simulink model "SimTest"  (R2019b)
settings: Solver=ode45  StartTime=0.0  StopTime=20  MaxStep=0.01  RelTol=1e-3  EnableMultiTasking=on
model workspace: external: MATLAB File sm_welding_robot_params.m (data not in the file)
values from neighbouring files (symbols this model uses):
  m = [6.25, 5, 1.25, 0.9817, 1.25, 0.125]    [ImprovedApproachLawSMC.m]    (also in Puma560CaneModel.m = [0, 17.4, 4.8, 0.82, 0.34, 0.09])
  N = N + m(i)*(cell2mat(W)*VT{i}'*(dVT{i}*cell2mat(WT')+VT{i}*cell2mat(dWT')))+W{i}*J{i}*dWT{i}+W{i}*WTdth{i}*J{i}*WT{i}    [ImprovedApproachLawSMC.m]    (also in Puma560CaneModel.m)
  s = c.*e + de    [ImprovedApproachLawSMC.m]
undefined symbols (not defined in the file or in its folder): color, density, path, robot, workpiece, X, Y, Z
libraries: sm_lib x63, nesl_utility x13, sm_welding_robot_lib x7
(part 1 of 2)
Description:
  | Computing Actuator Torques Using Inverse Dynamics
  | 
  | This example illustrates the use of motion actuation to determine the actuator torques needed for the robot to achieve a given welding task.
  | The system consists of a seven degree of freedom robot carrying a welding torch. The tip of the torch needs to trace the joints being welded. In
  | this example the tip of the torch is made to trace (using motion actuation) a plus sign, a circle and a star sign on the workpiece. The torch is
  | lifted off the workpiece when transitioning between the different shapes. The motion of the welding torch is specified and the actuator
  | torques required at the various joints of the robot to achieve this motion is computed.
settings Model: Creator=MathWorks  LastModifiedBy=Priscilla
settings DataIOCC: LimitDataPoints=on  SaveFormat=Array  SaveOutput=off  SaveTime=off  ReturnWorkspaceOutputs=off
settings OptimizationCC: LifeSpan=inf
settings DebuggingCC: UnderspecifiedInitializationDetection=Classic  MergeDetectMultiDrivingBlocksExec=none  SFUnexpectedBacktrackingDiag=warning  SFNoUnconditionalDefaultTransitionDiag=warning  SFExecutionAtInitializationDiag=none  ArithmeticOperatorsInVariantConditions=warning
settings HardwareCC: ProdBitPerPointer=32  ProdBitPerSizeT=32  ProdBitPerPtrDiffT=32  ProdLargestAtomicFloat=None  ProdIntDivRoundTo=Undefined  ProdEndianess=Unspecified  ProdWordSize=32  ProdHWDeviceType=32-bit Generic
settings ModelReferenceCC: PropagateSignalLabelsOutOfModel=off
settings SFSimCC: SimUseLocalCustomCode=off  CustomCodeUndefinedFunction=UseInterfaceOnly
settings RTWCC: RTWUseLocalCustomCode=off
settings CodeAppCC: StateflowObjectComments=on
settings GRTTargetCC: TargetLangStandard=C89/C90 (ANSI)  GeneratePreprocessorConditionals=Disable all
settings ConfigComp: CovMetricSettings=dw  CovHtmlReporting=on  CovSaveCumulativeToWorkspaceVar=on  CovSaveSingleToWorkspaceVar=on  CovExternalEMLEnable=off  CovSFcnEnable=off
settings SimscapeCC: SimscapeNormalizeSystem=off
settings ConfigurationSet: Description=SimMechanics 2G
settings DiagnosticsConfigSet: SimMechanicsUnconnectedFramePorts=none
settings ExplorerConfigSet: InternalSimMechanicsExplorerSettings="<ExplorerConfiguration><canonicalview>default</canonicalview><TilePanel><TileInfo><Tiles Columns=\"1\" Count=\"1\" Rows=\"1\"><Column Left=\"2\" Weight=\"1\"/><Column Left=\"702\"/><Row Top=\"2\" Weight=\"1\"/><Row Top=\"609\"/><Tile Height=\"1\" Width=\"1\" X=\"0\" Y=\"0\"/></Tiles></TileInfo><SceneInfo><SceneViewer><BGColor><R>0.60000002384185791</R><G>0.60000002384185791</G><B>0.60000002384185791</B></BGColor><Camera><Position><X>2.70313193911561722</X><Y>-2.01174652149009159</Y><Z>3.03337065647681836</Z></Position><Center><X>0.60321557915254076</X><Y>0.0881698384729807105</Y><Z>0.933454296513737347</Z></Center><Up><X>-0.408248290463863073</X><Y>0.408248290463863073</Y><Z>0.816496580927726145</Z></Up><Left>-0.59695774513732025</Left><Right>0.59695774513732025</Right><Bottom>-0.82465145012954455</Bottom><Top>0.82465145012954455</Top></Camera></SceneViewer></SceneInfo></TilePanel></ExplorerConfiguration>"

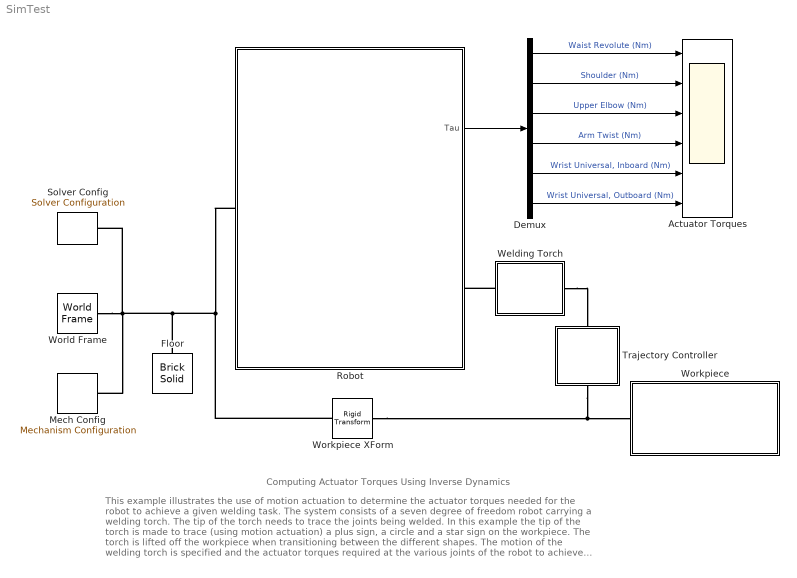
== system SimTest ==
  note: Computing Actuator Torques Using Inverse Dynamics
  note: This example illustrates the use of motion actuation to determine the actuator torques needed for the robot to achieve a given welding task.
      | The system consists of a seven degree of freedom robot carrying a welding torch. The tip of the torch needs to trace the joints being welded.
      | In this example the tip of the torch is made to trace (using motion actuation) a plus sign, a circle and a star sign on the workpiece. The torch is
      | lifted off the workpiece when transitioning between the different shapes. The motion of the welding torch is specified and the actuator torques
      | required at the various joints of the robot to achieve this motion are computed.
  Actuator Torques : Scope  NumInputPorts=6
  Demux : Demux  Outputs=6
  Floor : sm_lib/Body Elements/Brick Solid  GraphicAmbientColor=[0.15 0.15 0.15 1.0]  BasedOnType=Density  BrickDimensions=[floor.length floor.width floor.thickness]  BrickDimensionUnits=cm  CenterOfMass=[0 0 0]  CenterOfMassUnits=m  GraphicDiffuseColor=color.grey  Density=density.aluminum  DensityUnits=kg/(m^3)  DoExposeReferenceFrame=on  GraphicEmissiveColor=[0.0 0.0 0.0 1.0]  ExportEntireGeometry=off  SerializedFrames=<Frames/>  MarkerShape=Sphere  MarkerSize=10  GraphicType=FromGeometry  InertiaType=CalculateFromGeometry  Mass=1  MassUnits=kg  MomentsOfInertia=[1 1 1]  MomentsOfInertiaUnits=kg*m^2  GraphicOpacity=0.5  ProductsOfInertia=[0 0 0]  ProductsOfInertiaUnits=kg*m^2  GraphicShininess=75  GraphicSpecularColor=[0.5 0.5 0.5 1.0]  GraphicVisPropType=SimpleVisualProperties
  Mech Config : sm_lib/Utilities/Mechanism Configuration  UniformGravity=Constant  GravityVector=[0 0 -9.80665]  GravityUnits=m/s^2  LinearizationDelta=0.001
  Robot : Subsystem
      mask Display:
      | image(imread(fullfile(matlabroot,'toolbox','physmod','sm','smdemos','welding_robot','images','sm_wrobot_robot.png')));
      | port_label('RConn',1,'Tool')
      | port_label('LConn',1,'Floor')
      | port_label('output',1,'Tau')
  Solver Config : nesl_utility/Solver Configuration  PhysicalDomain=network_engine_domain  SubClassName=solver  LeftPortType=input  RightPortType=generic  Tones=[]  Harmonics=[]  SimulateNoise=off  Profile=off  UseLocalSampling=off  EnableSwitchedLinearOptims=on  FrequencyDomain=off  UseCCode=off  RelTol=0.001  AbsTol=1e-06  MinStep=1e-09  ToWorkspace=off  RevertToSquareIcSolve=off  NumHomotopyIterations=100  PhasorMode=off  PhasorModeNumHarmonics=1  DoDC=off  ResidualTolerance=1e-09  UseLocalSolver=off  LocalSolverChoice=NE_BACKWARD_EULER_ADVANCER  LocalSolverSampleTime=0.001  DoFixedCost=off  MaxNonlinIter=3  MaxModeIter=2  LinearAlgebra=Sparse  EquationFormulation=NE_TIME_EF  DelaysMemoryBudget=1024  AutomaticFiltering=on  FilteringTimeConstant=0.001  PartitionStorageMethod=AS_NEEDED  PartitionMemoryBudget=1024  PartitionMethod=FAST
  Trajectory Controller : Subsystem  mask(Trajectory Controller){tool_home=workpiece.tool.home, z_off=workpiece.tool.zoffset, glyph_sep=workpiece.glyphsep, plus_arm=workpiece.plus.armlength, circle_radius=workpiece.circle.radius, star_radius=workpiece.star.radius}
      mask prompts: tool_home "Tool Home (cm)"; z_off "Tool Off Distance (cm)"; glyph_sep "Glyph Separation (cm)"; plus_arm "Plus arm length (cm)"; circle_radius "Circle radius (cm)"; star_radius "Star circumcircle radius (cm)"
      mask help: This block controls the position and orientation of the follower frame (F) with respect to the base frame (B).
      mask init:
      | % Start tool path in home configuration
      | tool_path = [...
      |     0 tool_home'; ...
      |     1 tool_home'; ...
      |     ];
      | 
      | % Plus
      | plus = [ ...
      |     0   0 plus_arm/2 z_off; ...
      |     0.2 0 plus_arm/2 z_off; ...
      |     0.6 0 plus_arm/2 0; ...
      |     2.2 0 -plus_arm/2 0; ...
      |     2.6 -plus_arm/2 0 z_off; ...
      |     3   -plus_arm/2 0 0; ...
      |     4.6 +plus_arm/2 0 0; ...
      |     5   +plus_arm/2 0 z_off; ...
      |     ];
      | plus(:,2) = plus(:,2) - glyph_sep;
      | plus(:,1) = plus(:,1) + tool_path(end, 1) + 1;
      | tool_path = [tool_path; plus];
      | 
      | % Circle
      | dt = 3;
      | theta = (90:1:450)' * pi/180;
      | n = size(theta, 1);
      | pts = circle_radius * [cos(theta), sin(theta)];
      | circle = [ ...
      |     0 0 circle_radius z_off; ...
      |     linspace(0.4, 0.4 + dt, n)', pts, zeros(n, 1); ...
      |     (0.8 + dt) 0 circle_radius z_off; ...
      |     ];
      | circle(:,1) = circle(:,1) + tool_path(end, 1) + 1;
      | tool_path = [tool_path; circle];
      | 
      | % Star
      | dt = 3;
      | theta = (90:144:810)' * pi/180;
      | pts = star_radius * [cos(theta), sin(theta)];
      | star = [ ...
      |     0 0 star_radius z_off; ...
      |     linspace(0.4, 0.4 + dt, 6)', pts, zeros(6, 1); ...
      |     (0.8 + dt) 0 star_radius z_off; ...
      |     ];
      | star(:,2) = star(:,2) + glyph_sep;
      | star(:,1) = star(:,1) + tool_path(end, 1) + 1;
      | tool_path = [tool_path; star];
      | 
      | % End tool path in home configuration
      | home = [...
      |     0 tool_home'; ...
      |     1 tool_home'; ...
      |     ];
      | home(:,1) = home(:,1) + tool_path(end, 1) + 1;
      | tool_path = [tool_path; home];
      mask Display:
      | port_label('LConn',1,'B')
      | port_label('RConn',1,'F')
  Welding Torch : Subsystem  mask(Welding Torch){shaft_rad=robot.tool.shaftradius, length=robot.tool.length, tip_length=robot.tool.tiplength, tip_outer_rad=robot.tool.tiporadius, tip_inner_rad=robot.tool.tipiradius, density=density.aluminum, shaft_color=color.grey, tip_color=color.red}
      mask prompts: shaft_rad "Shaft Radius (cm)"; length "Tool Length (cm)"; tip_length "Tip Length (cm)"; tip_outer_rad "Tip Outer Radius (cm)"; tip_inner_rad "Tip Inner Radius (cm)"; density "Density (kg/m^3)"; shaft_color "Shaft Color (RGB)"; tip_color "Tip Color (RGB)"
      mask help:
      | This block models the welding torch.
      |
      | The port G corresponds to the base of the welding torch.
      |
      | The port T corresponds to the tip of the welding torch.
      mask init:
      | shaft_length = length - tip_length;
      | 
      | tip_cross_sect = [ ...
      |     0 0; ...
      |     tip_inner_rad 0;
      |     tip_outer_rad tip_length; ...
      |     0 tip_length ...
      |     ];
      mask DialogControl Container4 Prompt: Dimensions
      mask DialogControl Container4_copy Prompt: Material Properties
      mask Display:
      | image(imread(fullfile(matlabroot,'toolbox','physmod','sm','smdemos','welding_robot','images','sm_wrobot_tool.png')));
      | port_label('RConn',1,'T')
      | port_label('LConn',1,'G')
  Workpiece : Subsystem  mask(Workpiece){length=workpiece.plate.length, width=workpiece.plate.width, thickness=workpiece.plate.thickness, bead=workpiece.beadsize, plus_arm=workpiece.plus.armlength, circle_radius=workpiece.circle.radius, star_radius=workpiece.star.radius, density=density.aluminum, plate_color=color.lgreen, bead_color=color.dblue}
      mask prompts: length "Plate Length (cm)"; width "Plate Width (cm)"; thickness "Plate Thickness (cm)"; bead "Bead Size (cm)"; plus_arm "Plus arm length (cm)"; circle_radius "Circle radius (cm)"; star_radius "Star circumcircle radius (cm)"; density "Density (kg/m^3)"; plate_color "Plate Color (RGB)"; bead_color "Bead Color (RGB)"
      mask help:
      | This block models a rectangular workpiece with three different shapes engraved on it. A plus sign, a circle and a star are engraved on the workpiece. The robot tool tip is expected to track the engraved shapes.
      |
      | The port R corresponds to the frame at the center of the workpiece.
      mask DialogControl Container4 Prompt: Dimensions
      mask DialogControl Container5 Prompt: Material Properties
      mask Display:
      | image(imread(fullfile(matlabroot,'toolbox','physmod','sm','smdemos','welding_robot','images','sm_wrobot_workpiece.png')));
      | port_label('LConn',1,'R')
  Workpiece XForm : sm_lib/Frames and Transforms/Rigid Transform  TranslationMethod=Cartesian  TranslationStandardOffset=0  TranslationLengthUnit=cm  TranslationStandardAxis=+Z  TranslationCartesianOffset=[workpiece.distance 0 workpiece.height]  TranslationROffset=0  TranslationROffsetUnits=m  TranslationZOffset=0  TranslationZOffsetUnits=m  TranslationThetaOffset=0  TranslationThetaOffsetUnits=deg  RotationMethod=AlignedAxes  RotationAngleUnits=deg  RotationStandardAxis=+Z  RotationAngle=0  RotationArbitraryAxis=[0 0 1]  FollAlignAxisA=+Z  BaseAlignAxisA=-X  FollAlignAxisB=+Y  BaseAlignAxisB=+Z  RotationSequenceAxes=FollowerAxes  RotationSequence=XYX  RotationSequenceAngles=[0 0 0]  RotationSequenceAnglesUnits=deg  RotationMatrix=[1 0 0; 0 1 0; 0 0 1]
  World Frame : sm_lib/Frames and Transforms/World Frame
  wires:
  Demux/4 -> Actuator Torques/4  "Arm Twist (Nm)"
  Demux/1 -> Actuator Torques/1  "Waist Revolute (Nm)"
  Demux/2 -> Actuator Torques/2  "Shoulder (Nm)"
  Demux/3 -> Actuator Torques/3  "Upper Elbow (Nm)"
  Demux/5 -> Actuator Torques/5  "Wrist Universal, Inboard (Nm)"
  Demux/6 -> Actuator Torques/6  "Wrist Universal, Outboard (Nm)"
  Robot/1(Tau) -> Demux/1
  connections:
  Mech Config/RConn1 -- Floor/RConn1 -- Robot/LConn1 -- Workpiece XForm/LConn1 -- Solver Config/RConn1 -- World Frame/RConn1
  Trajectory Controller/LConn1 -- Workpiece XForm/RConn1 -- Workpiece/LConn1
  Welding Torch/LConn1 -- Robot/RConn1
  Welding Torch/RConn1 -- Trajectory Controller/RConn1

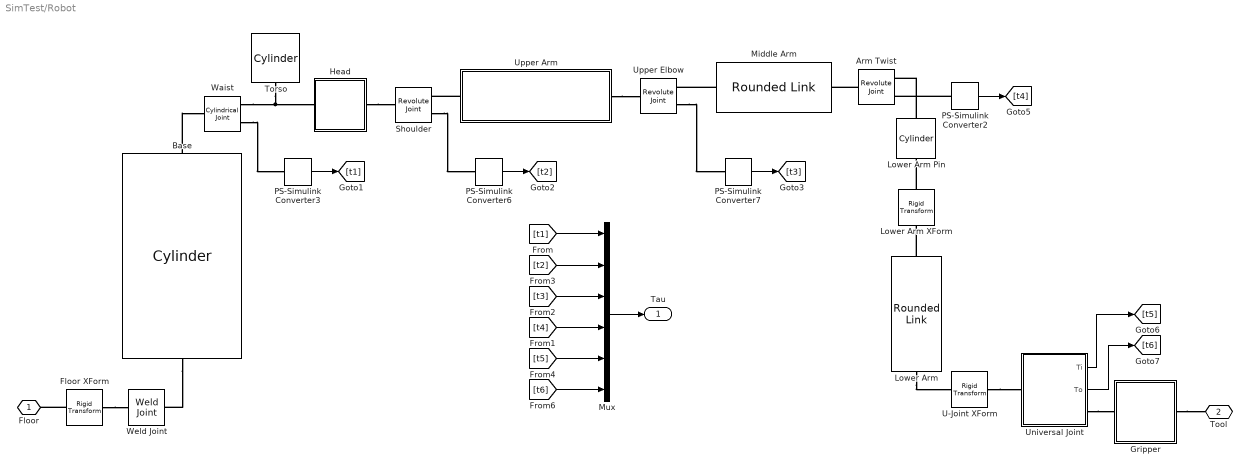
== system SimTest/Robot ==
  Arm Twist : sm_lib/Joints/Revolute Joint  JointMode=Normal  SenseConstraintForce=off  SenseConstraintForceX=off  SenseConstraintForceY=off  SenseConstraintForceZ=off  SenseConstraintTorque=off  SenseConstraintTorqueX=off  SenseConstraintTorqueY=off  SenseConstraintTorqueZ=off  SenseTotalForce=off  SenseTotalForceX=off  SenseTotalForceY=off  SenseTotalForceZ=off  SenseTotalTorque=off  SenseTotalTorqueX=off  SenseTotalTorqueY=off  SenseTotalTorqueZ=off  CompositeWrenchDir=FollowerOnBase  CompositeWrenchFrame=BaseFrame  EquilibriumPosition=0  EquilibriumPositionUnits=deg  SpringStiffness=0  SpringStiffnessUnits=N*m/deg  DampingCoefficient=0  DampingCoefficientUnits=N*m/(deg/s)  TorqueActuationMode=ComputedTorque  MotionActuationMode=ComputedMotion  SensePosition=off  SenseVelocity=off  SenseAcceleration=off  SenseTorqueForce=on  SenseLowerLimitTorqueForce=off  SenseUpperLimitTorqueForce=off  LowerLimitSpecify=off  LowerLimitBound=-90  LowerLimitBoundUnits=deg  LowerLimitStiffness=1e4  LowerLimitStiffnessUnits=N*m/deg  LowerLimitDamping=10  LowerLimitDampingUnits=N*m/(deg/s)  LowerLimitTransitionRegionWidth=0.1  LowerLimitTransitionRegionWidthUnits=deg  UpperLimitSpecify=off  UpperLimitBound=90  UpperLimitBoundUnits=deg  UpperLimitStiffness=1e4  UpperLimitStiffnessUnits=N*m/deg  UpperLimitDamping=10  UpperLimitDampingUnits=N*m/(deg/s)  UpperLimitTransitionRegionWidth=0.1  UpperLimitTransitionRegionWidthUnits=deg  PositionTargetSpecify=on  PositionTargetPriority=High  PositionTargetValue=0  PositionTargetValueUnits=deg  VelocityTargetSpecify=off  VelocityTargetPriority=High  VelocityTargetValue=0  VelocityTargetValueUnits=deg/s
  Base : sm_welding_robot_lib/Cylinder  radius=robot.base.radius  length=robot.base.height  density=density.aluminum  color=color.dblue
      settings: SourceProductName=Simscape Multibody  SourceProductBaseCode=MS
  Floor XForm : sm_lib/Frames and Transforms/Rigid Transform  TranslationMethod=StandardAxis  TranslationStandardOffset=floor.thickness/2  TranslationLengthUnit=cm  TranslationStandardAxis=+Z  TranslationCartesianOffset=[0 0 0.02]  TranslationROffset=0  TranslationROffsetUnits=m  TranslationZOffset=0  TranslationZOffsetUnits=m  TranslationThetaOffset=0  TranslationThetaOffsetUnits=deg  RotationMethod=None  RotationAngleUnits=deg  RotationStandardAxis=+Z  RotationAngle=0  RotationArbitraryAxis=[0 0 1]  FollAlignAxisA=+X  BaseAlignAxisA=+Y  FollAlignAxisB=+Y  BaseAlignAxisB=+Z  RotationSequenceAxes=FollowerAxes  RotationSequence=XYX  RotationSequenceAngles=[0 0 0]  RotationSequenceAnglesUnits=deg  RotationMatrix=[1 0 0; 0 1 0; 0 0 1]
  Gripper : Subsystem  mask(Gripper){base_rad=robot.gripper.baseradius, base_thickness=robot.gripper.basethickness, tip_rad=robot.gripper.tipradius, tip_depth=robot.gripper.tipdepth, claw_length=robot.gripper.clawlength, tool_rad=robot.gripper.channelradius, density=density.aluminum, color=color.lblue}
      mask prompts: base_rad "Base Radius (mm)"; base_thickness "Base Thickness (mm)"; tip_rad "Tip Radius (mm)"; tip_depth "Tip Depth (mm)"; claw_length "Claw Length (mm)"; tool_rad "Tool Channel Radius (mm)"; density "Density (kg/m^3)"; color "Color (RGB)"
      mask help:
      | This block models a gripper with four claws.
      |
      | The port B refers to the frame at the center of the bottom face of the gripper base.
      |
      | The port T refers to the frame at the center of the top face of the gripper base.
      mask init:
      | claw_cross_sect = [ ...
      |     (tool_rad + base_rad) / 2, 0; ...
      |     base_rad * 0.9, 0; ...
      |     tip_rad, claw_length; ...
      |     tool_rad, claw_length; ...
      |     tool_rad, claw_length - tip_depth ...
      |     ];
      mask DialogControl Container4 Prompt: Dimensions
      mask DialogControl Container5 Prompt: Material Properties
      mask Display:
      | image(imread(fullfile(matlabroot,'toolbox','physmod','sm','smdemos','welding_robot','images','sm_wrobot_gripper.png')));
      | port_label('RConn',1,'T')
      | port_label('LConn',1,'B')
  Head : Subsystem  mask(Cube){length=robot.head.length, width=robot.head.width, height=robot.head.height, shoulder_offset=robot.shoulder.offset, density=density.aluminum, color=color.lblue}
      mask prompts: length "Length (cm)"; width "Width (cm)"; height "Height (cm)"; shoulder_offset "Shoulder Offset (cm)"; density "Density (kg/m^3)"; color "Color (rgb)"
      mask help: This block models a cube with a frame at the base face (T) and side face (A) of the cube.
      mask DialogControl Container4 Prompt: Dimensions
      mask DialogControl Container4_copy Prompt: Material Properties
      mask Display:
      | image(imread(fullfile(matlabroot,'toolbox','physmod','sm','smdemos','welding_robot','images','sm_wrobot_head.png')));
      | port_label('RConn',1,'A')
      | port_label('LConn',1,'T')
  Lower Arm Pin : sm_welding_robot_lib/Cylinder  radius=robot.lowerarmpin.radius  length=robot.lowerarmpin.height  density=density.aluminum  color=color.brown
      settings: SourceProductName=Simscape Multibody  SourceProductBaseCode=MS
  Lower Arm : sm_welding_robot_lib/Rounded Link  length=robot.lowerarm.length  rad_in=robot.lowerarm.radius  flatwidth=robot.lowerarm.width  thickness=robot.lowerarm.thickness  color=color.yellow  density=density.aluminum
      settings: SourceProductName=Simscape Multibody  SourceProductBaseCode=MS
  Lower Arm XForm : sm_lib/Frames and Transforms/Rigid Transform  TranslationMethod=None  TranslationStandardOffset=0  TranslationLengthUnit=m  TranslationStandardAxis=+Z  TranslationCartesianOffset=[0 0 0]  TranslationROffset=0  TranslationROffsetUnits=m  TranslationZOffset=0  TranslationZOffsetUnits=m  TranslationThetaOffset=0  TranslationThetaOffsetUnits=deg  RotationMethod=AlignedAxes  RotationAngleUnits=deg  RotationStandardAxis=+Z  RotationAngle=0  RotationArbitraryAxis=[0 0 1]  FollAlignAxisA=+Z  BaseAlignAxisA=-Z  FollAlignAxisB=+X  BaseAlignAxisB=+X  RotationSequenceAxes=FollowerAxes  RotationSequence=XYX  RotationSequenceAngles=[0 0 0]  RotationSequenceAnglesUnits=deg  RotationMatrix=[1 0 0; 0 1 0; 0 0 1]
  Middle Arm : sm_welding_robot_lib/Rounded Link  length=robot.middlearm.length  rad_in=robot.middlearm.radius  flatwidth=robot.middlearm.width  thickness=robot.middlearm.thickness  color=color.lbrown  density=density.aluminum
      settings: SourceProductName=Simscape Multibody  SourceProductBaseCode=MS
  Mux : Mux  Inputs=6
  PS-Simulink Converter{2..3,6..7} (4 alike) : nesl_utility/PS-Simulink Converter  PhysicalDomain=network_engine_domain  SubClassName=ps_output  LeftPortType=input  RightPortType=output  PseudoPeriodic=off  Frequencies=[]  Unit=N*m  AffineConversion=off
  Shoulder : sm_lib/Joints/Revolute Joint  JointMode=Normal  SenseConstraintForce=off  SenseConstraintForceX=off  SenseConstraintForceY=off  SenseConstraintForceZ=off  SenseConstraintTorque=off  SenseConstraintTorqueX=off  SenseConstraintTorqueY=off  SenseConstraintTorqueZ=off  SenseTotalForce=off  SenseTotalForceX=off  SenseTotalForceY=off  SenseTotalForceZ=off  SenseTotalTorque=off  SenseTotalTorqueX=off  SenseTotalTorqueY=off  SenseTotalTorqueZ=off  CompositeWrenchDir=FollowerOnBase  CompositeWrenchFrame=BaseFrame  EquilibriumPosition=0  EquilibriumPositionUnits=deg  SpringStiffness=0  SpringStiffnessUnits=N*m/deg  DampingCoefficient=0  DampingCoefficientUnits=N*m/(deg/s)  TorqueActuationMode=ComputedTorque  MotionActuationMode=ComputedMotion  SensePosition=off  SenseVelocity=off  SenseAcceleration=off  SenseTorqueForce=on  SenseLowerLimitTorqueForce=off  SenseUpperLimitTorqueForce=off  LowerLimitSpecify=off  LowerLimitBound=-90  LowerLimitBoundUnits=deg  LowerLimitStiffness=1e4  LowerLimitStiffnessUnits=N*m/deg  LowerLimitDamping=10  LowerLimitDampingUnits=N*m/(deg/s)  LowerLimitTransitionRegionWidth=0.1  LowerLimitTransitionRegionWidthUnits=deg  UpperLimitSpecify=off  UpperLimitBound=90  UpperLimitBoundUnits=deg  UpperLimitStiffness=1e4  UpperLimitStiffnessUnits=N*m/deg  UpperLimitDamping=10  UpperLimitDampingUnits=N*m/(deg/s)  UpperLimitTransitionRegionWidth=0.1  UpperLimitTransitionRegionWidthUnits=deg  PositionTargetSpecify=on  PositionTargetPriority=Low  PositionTargetValue=0  PositionTargetValueUnits=deg  VelocityTargetSpecify=off  VelocityTargetPriority=High  VelocityTargetValue=0  VelocityTargetValueUnits=deg/s
  Torso : sm_welding_robot_lib/Cylinder  radius=robot.torso.radius  length=robot.torso.height  density=density.aluminum  color=color.lblue
      settings: SourceProductName=Simscape Multibody  SourceProductBaseCode=MS
  U-Joint XForm : sm_lib/Frames and Transforms/Rigid Transform  TranslationMethod=None  TranslationStandardOffset=5  TranslationLengthUnit=cm  TranslationStandardAxis=+X  TranslationCartesianOffset=[0 0 0]  TranslationROffset=0  TranslationROffsetUnits=m  TranslationZOffset=0  TranslationZOffsetUnits=m  TranslationThetaOffset=0  TranslationThetaOffsetUnits=deg  RotationMethod=AlignedAxes  RotationAngleUnits=deg  RotationStandardAxis=+Z  RotationAngle=0  RotationArbitraryAxis=[0 0 1]  FollAlignAxisA=+Z  BaseAlignAxisA=-X  FollAlignAxisB=+Y  BaseAlignAxisB=+Y  RotationSequenceAxes=FollowerAxes  RotationSequence=XYX  RotationSequenceAngles=[0 0 0]  RotationSequenceAnglesUnits=deg  RotationMatrix=[1 0 0; 0 1 0; 0 0 1]
  Universal Joint : Subsystem
      mask Display:
      | image(imread(fullfile(matlabroot,'toolbox','physmod','sm','smdemos','welding_robot','images','sm_wrobot_univjoint.png')));
      | port_label('RConn',1,'G')
      | port_label('LConn',1,'LA')
      | port_label('output',1,'Ti')
      | port_label('output',2,'To')
  Upper Arm : Subsystem  mask(Rounded Tapered Link){length=robot.upperarm.length, rad_in=robot.upperarm.iradius, thickness=robot.upperarm.thickness, rad_out=robot.upperarm.oradius, density=density.aluminum, color=color.orange}
      mask prompts: length "Length (cm)"; rad_in "Inboard Radius (cm)"; thickness "Thickness (cm)"; rad_out "Outboard Radius (cm)"; density "Density (kg/m^3)"; color "Color (rgb)"
      mask help:
      | This block models a link that has two rounded ends (inboard and outboard).The link tapers from the inboard to outboard end.
      |
      | The two ports correspond to the frames at the centers of the inboard (I) and outboard (O) rounded sections.
      mask init:
      | theta_in = (pi/2:0.01:3*pi/2)';
      | arc_in = rad_in * [cos(theta_in), sin(theta_in)];
      | 
      | theta_out = (-pi/2:0.01:+pi/2)';
      | arc_out = rad_out * [cos(theta_out), sin(theta_out)] ...
      |     + repmat([length 0], size(theta_out));
      | 
      | cross_sect = [arc_in; arc_out];
      mask DialogControl Container4 Prompt: Dimensions
      mask DialogControl Container4_copy Prompt: Material Properties
      mask Display:
      | image(imread(fullfile(matlabroot,'toolbox','physmod','sm','smdemos','welding_robot','images','sm_wrobot_upperarm.png')));
      | port_label('RConn',1,'O')
      | port_label('LConn',1,'I')
  Upper Elbow : sm_lib/Joints/Revolute Joint  JointMode=Normal  SenseConstraintForce=off  SenseConstraintForceX=off  SenseConstraintForceY=off  SenseConstraintForceZ=off  SenseConstraintTorque=off  SenseConstraintTorqueX=off  SenseConstraintTorqueY=off  SenseConstraintTorqueZ=off  SenseTotalForce=off  SenseTotalForceX=off  SenseTotalForceY=off  SenseTotalForceZ=off  SenseTotalTorque=off  SenseTotalTorqueX=off  SenseTotalTorqueY=off  SenseTotalTorqueZ=off  CompositeWrenchDir=FollowerOnBase  CompositeWrenchFrame=BaseFrame  EquilibriumPosition=0  EquilibriumPositionUnits=deg  SpringStiffness=0  SpringStiffnessUnits=N*m/deg  DampingCoefficient=0  DampingCoefficientUnits=N*m/(deg/s)  TorqueActuationMode=ComputedTorque  MotionActuationMode=ComputedMotion  SensePosition=off  SenseVelocity=off  SenseAcceleration=off  SenseTorqueForce=on  SenseLowerLimitTorqueForce=off  SenseUpperLimitTorqueForce=off  LowerLimitSpecify=off  LowerLimitBound=-90  LowerLimitBoundUnits=deg  LowerLimitStiffness=1e4  LowerLimitStiffnessUnits=N*m/deg  LowerLimitDamping=10  LowerLimitDampingUnits=N*m/(deg/s)  LowerLimitTransitionRegionWidth=0.1  LowerLimitTransitionRegionWidthUnits=deg  UpperLimitSpecify=off  UpperLimitBound=90  UpperLimitBoundUnits=deg  UpperLimitStiffness=1e4  UpperLimitStiffnessUnits=N*m/deg  UpperLimitDamping=10  UpperLimitDampingUnits=N*m/(deg/s)  UpperLimitTransitionRegionWidth=0.1  UpperLimitTransitionRegionWidthUnits=deg  PositionTargetSpecify=on  PositionTargetPriority=Low  PositionTargetValue=90  PositionTargetValueUnits=deg  VelocityTargetSpecify=off  VelocityTargetPriority=High  VelocityTargetValue=0  VelocityTargetValueUnits=deg/s
  Waist : sm_lib/Joints/Cylindrical Joint  JointMode=Normal  SenseConstraintForce=off  SenseConstraintForceX=off  SenseConstraintForceY=off  SenseConstraintForceZ=off  SenseConstraintTorque=off  SenseConstraintTorqueX=off  SenseConstraintTorqueY=off  SenseConstraintTorqueZ=off  SenseTotalForce=off  SenseTotalForceX=off  SenseTotalForceY=off  SenseTotalForceZ=off  SenseTotalTorque=off  SenseTotalTorqueX=off  SenseTotalTorqueY=off  SenseTotalTorqueZ=off  CompositeWrenchDir=FollowerOnBase  CompositeWrenchFrame=BaseFrame  PzEquilibriumPosition=10  PzEquilibriumPositionUnits=cm  PzSpringStiffness=400  PzSpringStiffnessUnits=N/cm  PzDampingCoefficient=20  PzDampingCoefficientUnits=N/(cm/s)  PzTorqueActuationMode=NoTorque  PzMotionActuationMode=ComputedMotion  PzSensePosition=off  PzSenseVelocity=off  PzSenseAcceleration=off  PzSenseTorqueForce=off  PzSenseLowerLimitTorqueForce=off  PzSenseUpperLimitTorqueForce=off  PzLowerLimitSpecify=off  PzLowerLimitBound=-1  PzLowerLimitBoundUnits=m  PzLowerLimitStiffness=1e6  PzLowerLimitStiffnessUnits=N/m  PzLowerLimitDamping=1e3  PzLowerLimitDampingUnits=N/(m/s)  PzLowerLimitTransitionRegionWidth=1e-4  PzLowerLimitTransitionRegionWidthUnits=m  PzUpperLimitSpecify=off  PzUpperLimitBound=1  PzUpperLimitBoundUnits=m  PzUpperLimitStiffness=1e6  PzUpperLimitStiffnessUnits=N/m  PzUpperLimitDamping=1e3  PzUpperLimitDampingUnits=N/(m/s)  PzUpperLimitTransitionRegionWidth=1e-4  PzUpperLimitTransitionRegionWidthUnits=m  PzPositionTargetSpecify=on  PzPositionTargetPriority=High  PzPositionTargetValue=10  PzPositionTargetValueUnits=cm  PzVelocityTargetSpecify=off  PzVelocityTargetPriority=High  PzVelocityTargetValue=0  PzVelocityTargetValueUnits=m/s  RzEquilibriumPosition=0  RzEquilibriumPositionUnits=deg  RzSpringStiffness=0  RzSpringStiffnessUnits=N*m/deg  RzDampingCoefficient=0  RzDampingCoefficientUnits=N*m/(deg/s)  RzTorqueActuationMode=ComputedTorque  RzMotionActuationMode=ComputedMotion  RzSensePosition=off  RzSenseVelocity=off  RzSenseAcceleration=off  RzSenseTorqueForce=on  RzSenseLowerLimitTorqueForce=off  RzSenseUpperLimitTorqueForce=off  RzLowerLimitSpecify=off  RzLowerLimitBound=-90  RzLowerLimitBoundUnits=deg  RzLowerLimitStiffness=1e4  RzLowerLimitStiffnessUnits=N*m/deg  RzLowerLimitDamping=10  RzLowerLimitDampingUnits=N*m/(deg/s)  RzLowerLimitTransitionRegionWidth=0.1  RzLowerLimitTransitionRegionWidthUnits=deg  RzUpperLimitSpecify=off  RzUpperLimitBound=90  RzUpperLimitBoundUnits=deg  RzUpperLimitStiffness=1e4  RzUpperLimitStiffnessUnits=N*m/deg  RzUpperLimitDamping=10  RzUpperLimitDampingUnits=N*m/(deg/s)  RzUpperLimitTransitionRegionWidth=0.1  RzUpperLimitTransitionRegionWidthUnits=deg  RzPositionTargetSpecify=on  RzPositionTargetPriority=Low  RzPositionTargetValue=0  RzPositionTargetValueUnits=deg  RzVelocityTargetSpecify=off  RzVelocityTargetPriority=High  RzVelocityTargetValue=0  RzVelocityTargetValueUnits=deg/s
  Weld Joint : sm_lib/Joints/Weld Joint  JointMode=Normal  SenseConstraintForce=off  SenseConstraintForceX=off  SenseConstraintForceY=off  SenseConstraintForceZ=off  SenseConstraintTorque=off  SenseConstraintTorqueX=off  SenseConstraintTorqueY=off  SenseConstraintTorqueZ=off  SenseTotalForce=off  SenseTotalForceX=off  SenseTotalForceY=off  SenseTotalForceZ=off  SenseTotalTorque=off  SenseTotalTorqueX=off  SenseTotalTorqueY=off  SenseTotalTorqueZ=off  CompositeWrenchDir=FollowerOnBase  CompositeWrenchFrame=BaseFrame
  Floor : PMIOPort  Side=Left
  Tool : PMIOPort  Port=2  Side=Right
  Tau : Outport  VectorParamsAs1DForOutWhenUnconnected=off
  wires:
  PS-Simulink Converter3/1 -> [t1]
  PS-Simulink Converter6/1 -> [t2]
  PS-Simulink Converter7/1 -> [t3]
  Universal Joint/1(Ti) -> [t5]
  Universal Joint/2(To) -> [t6]
  [t1] -> Mux/1
  [t2] -> Mux/2
  [t4] -> Mux/4
  [t5] -> Mux/5
  [t3] -> Mux/3
  Mux/1 -> Tau/1
  PS-Simulink Converter2/1 -> [t4]
  [t6] -> Mux/6
  connections:
  Head/RConn1 -- Shoulder/LConn1
  Waist/RConn1 -- Torso/RConn1 -- Head/LConn1
  Base/RConn1 -- Waist/LConn1
  Upper Arm/RConn1 -- Upper Elbow/LConn1
  Upper Arm/LConn1 -- Shoulder/RConn1
  U-Joint XForm/RConn1 -- Universal Joint/LConn1
  Universal Joint/RConn1 -- Gripper/LConn1
  Gripper/RConn1 -- Tool/RConn1
  Base/LConn1 -- Weld Joint/RConn1
  Shoulder/RConn2 -- PS-Simulink Converter6/LConn1
  Upper Elbow/RConn2 -- PS-Simulink Converter7/LConn1
  Waist/RConn2 -- PS-Simulink Converter3/LConn1
  Middle Arm/LConn1 -- Upper Elbow/RConn1
  Arm Twist/LConn1 -- Middle Arm/RConn1
  Lower Arm/LConn1 -- U-Joint XForm/LConn1
  PS-Simulink Converter2/LConn1 -- Arm Twist/RConn2
  Lower Arm Pin/LConn1 -- Arm Twist/RConn1
  Lower Arm XForm/LConn1 -- Lower Arm Pin/RConn1
  Lower Arm/RConn1 -- Lower Arm XForm/RConn1
  Floor XForm/RConn1 -- Weld Joint/LConn1
  Floor XForm/LConn1 -- Floor/RConn1

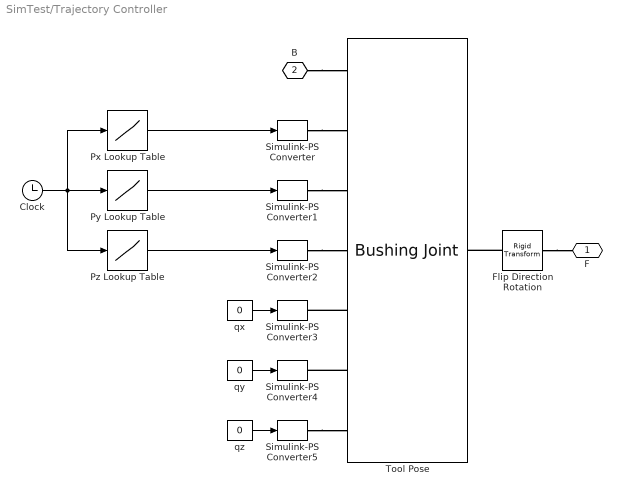
== system SimTest/Trajectory Controller ==
  Clock : Clock
  Flip Direction Rotation : sm_lib/Frames and Transforms/Rigid Transform  TranslationMethod=None  TranslationStandardOffset=0  TranslationLengthUnit=m  TranslationStandardAxis=+Z  TranslationCartesianOffset=[0 0 0]  TranslationROffset=0  TranslationROffsetUnits=m  TranslationZOffset=0  TranslationZOffsetUnits=m  TranslationThetaOffset=0  TranslationThetaOffsetUnits=deg  RotationMethod=AlignedAxes  RotationAngleUnits=deg  RotationStandardAxis=+Z  RotationAngle=0  RotationArbitraryAxis=[0 0 1]  FollAlignAxisA=+Z  BaseAlignAxisA=-Z  FollAlignAxisB=+Y  BaseAlignAxisB=+X  RotationSequenceAxes=FollowerAxes  RotationSequence=XYX  RotationSequenceAngles=[0 0 0]  RotationSequenceAnglesUnits=deg  RotationMatrix=[1 0 0; 0 1 0; 0 0 1]
  Px Lookup Table : Lookup_n-D  NumberOfTableDimensions=1  BreakpointsForDimension1=tool_path(:, 1)  BreakpointsForDimension2=[2 3 4]  BreakpointsForDimension3=path(:, 1)  BeginIndexSearchUsingPreviousIndexResult=on  Table=tool_path(:, 2)  RndMeth=Simplest
  Py Lookup Table : Lookup_n-D  NumberOfTableDimensions=1  BreakpointsForDimension1=tool_path(:, 1)  Table=tool_path(:, 3)  RndMeth=Simplest  InputSameDT=on
  Pz Lookup Table : Lookup_n-D  NumberOfTableDimensions=1  BreakpointsForDimension1=tool_path(:, 1)  Table=tool_path(:, 4)  RndMeth=Simplest  InputSameDT=on
  Simulink-PS Converter : nesl_utility/Simulink-PS Converter  PhysicalDomain=network_engine_domain  SubClassName=ps_input  LeftPortType=input  RightPortType=output  PseudoPeriodic=off  Frequencies=[]  NoiseDistribution=none  NoiseParameters=[]  Unit=cm  AffineConversion=off  FilteringAndDerivatives=filter  SimscapeFilterOrder=2  InputFilterTimeConstant=motion_tc  UdotUserProvided=1
  Simulink-PS Converter1 : nesl_utility/Simulink-PS Converter  PhysicalDomain=network_engine_domain  SubClassName=ps_input  LeftPortType=input  RightPortType=output  PseudoPeriodic=off  Frequencies=[]  NoiseDistribution=none  NoiseParameters=[]  Unit=cm  AffineConversion=off  FilteringAndDerivatives=filter  SimscapeFilterOrder=2  InputFilterTimeConstant=motion_tc  UdotUserProvided=1
  Simulink-PS Converter2 : nesl_utility/Simulink-PS Converter  PhysicalDomain=network_engine_domain  SubClassName=ps_input  LeftPortType=input  RightPortType=output  PseudoPeriodic=off  Frequencies=[]  NoiseDistribution=none  NoiseParameters=[]  Unit=cm  AffineConversion=off  FilteringAndDerivatives=filter  SimscapeFilterOrder=2  InputFilterTimeConstant=motion_tc  UdotUserProvided=1
  Simulink-PS Converter3 : nesl_utility/Simulink-PS Converter  PhysicalDomain=network_engine_domain  SubClassName=ps_input  LeftPortType=input  RightPortType=output  PseudoPeriodic=off  Frequencies=[]  NoiseDistribution=none  NoiseParameters=[]  Unit=deg  AffineConversion=off  FilteringAndDerivatives=filter  SimscapeFilterOrder=2  InputFilterTimeConstant=motion_tc  UdotUserProvided=1
  Simulink-PS Converter4 : nesl_utility/Simulink-PS Converter  PhysicalDomain=network_engine_domain  SubClassName=ps_input  LeftPortType=input  RightPortType=output  PseudoPeriodic=off  Frequencies=[]  NoiseDistribution=none  NoiseParameters=[]  Unit=deg  AffineConversion=off  FilteringAndDerivatives=filter  SimscapeFilterOrder=2  InputFilterTimeConstant=motion_tc  UdotUserProvided=1
  Simulink-PS Converter5 : nesl_utility/Simulink-PS Converter  PhysicalDomain=network_engine_domain  SubClassName=ps_input  LeftPortType=input  RightPortType=output  PseudoPeriodic=off  Frequencies=[]  NoiseDistribution=none  NoiseParameters=[]  Unit=deg  AffineConversion=off  FilteringAndDerivatives=filter  SimscapeFilterOrder=2  InputFilterTimeConstant=motion_tc  UdotUserProvided=1
  Tool Pose : sm_lib/Joints/Bushing Joint  JointMode=Normal  SenseConstraintForce=off  SenseConstraintForceX=off  SenseConstraintForceY=off  SenseConstraintForceZ=off  SenseConstraintTorque=off  SenseConstraintTorqueX=off  SenseConstraintTorqueY=off  SenseConstraintTorqueZ=off  SenseTotalForce=off  SenseTotalForceX=off  SenseTotalForceY=off  SenseTotalForceZ=off  SenseTotalTorque=off  SenseTotalTorqueX=off  SenseTotalTorqueY=off  SenseTotalTorqueZ=off  CompositeWrenchDir=FollowerOnBase  CompositeWrenchFrame=BaseFrame  PxEquilibriumPosition=0  PxEquilibriumPositionUnits=m  PxSpringStiffness=0  PxSpringStiffnessUnits=N/m  PxDampingCoefficient=0  PxDampingCoefficientUnits=N/(m/s)  PxTorqueActuationMode=NoTorque  PxMotionActuationMode=InputMotion  PxSensePosition=off  PxSenseVelocity=off  PxSenseAcceleration=off  PxSenseTorqueForce=off  PxSenseLowerLimitTorqueForce=off  PxSenseUpperLimitTorqueForce=off  PxLowerLimitSpecify=off  PxLowerLimitBound=-1  PxLowerLimitBoundUnits=m  PxLowerLimitStiffness=1e6  PxLowerLimitStiffnessUnits=N/m  PxLowerLimitDamping=1e3  PxLowerLimitDampingUnits=N/(m/s)  PxLowerLimitTransitionRegionWidth=1e-4  PxLowerLimitTransitionRegionWidthUnits=m  PxUpperLimitSpecify=off  PxUpperLimitBound=1  PxUpperLimitBoundUnits=m  PxUpperLimitStiffness=1e6  PxUpperLimitStiffnessUnits=N/m  PxUpperLimitDamping=1e3  PxUpperLimitDampingUnits=N/(m/s)  PxUpperLimitTransitionRegionWidth=1e-4  PxUpperLimitTransitionRegionWidthUnits=m  PxPositionTargetSpecify=off  PxPositionTargetPriority=High  PxPositionTargetValue=0  PxPositionTargetValueUnits=m  PxVelocityTargetSpecify=off  PxVelocityTargetPriority=High  PxVelocityTargetValue=0  PxVelocityTargetValueUnits=m/s  PyEquilibriumPosition=0  PyEquilibriumPositionUnits=m  PySpringStiffness=0  PySpringStiffnessUnits=N/m  PyDampingCoefficient=0  PyDampingCoefficientUnits=N/(m/s)  PyTorqueActuationMode=NoTorque  PyMotionActuationMode=InputMotion  PySensePosition=off  PySenseVelocity=off  PySenseAcceleration=off  PySenseTorqueForce=off  PySenseLowerLimitTorqueForce=off  PySenseUpperLimitTorqueForce=off  PyLowerLimitSpecify=off  PyLowerLimitBound=-1  PyLowerLimitBoundUnits=m  PyLowerLimitStiffness=1e6  PyLowerLimitStiffnessUnits=N/m  PyLowerLimitDamping=1e3  PyLowerLimitDampingUnits=N/(m/s)  PyLowerLimitTransitionRegionWidth=1e-4  PyLowerLimitTransitionRegionWidthUnits=m  PyUpperLimitSpecify=off  PyUpperLimitBound=1  PyUpperLimitBoundUnits=m  PyUpperLimitStiffness=1e6  PyUpperLimitStiffnessUnits=N/m  PyUpperLimitDamping=1e3  PyUpperLimitDampingUnits=N/(m/s)  PyUpperLimitTransitionRegionWidth=1e-4  PyUpperLimitTransitionRegionWidthUnits=m  PyPositionTargetSpecify=off  PyPositionTargetPriority=High  PyPositionTargetValue=0  PyPositionTargetValueUnits=m  PyVelocityTargetSpecify=off  PyVelocityTargetPriority=High  PyVelocityTargetValue=0  PyVelocityTargetValueUnits=m/s  PzEquilibriumPosition=0  PzEquilibriumPositionUnits=m  PzSpringStiffness=0  PzSpringStiffnessUnits=N/m  PzDampingCoefficient=0  PzDampingCoefficientUnits=N/(m/s)  PzTorqueActuationMode=NoTorque  PzMotionActuationMode=InputMotion  PzSensePosition=off  PzSenseVelocity=off  PzSenseAcceleration=off  PzSenseTorqueForce=off  PzSenseLowerLimitTorqueForce=off  PzSenseUpperLimitTorqueForce=off  PzLowerLimitSpecify=off  PzLowerLimitBound=-1  PzLowerLimitBoundUnits=m  PzLowerLimitStiffness=1e6  PzLowerLimitStiffnessUnits=N/m  PzLowerLimitDamping=1e3  PzLowerLimitDampingUnits=N/(m/s)  PzLowerLimitTransitionRegionWidth=1e-4  PzLowerLimitTransitionRegionWidthUnits=m  PzUpperLimitSpecify=off  PzUpperLimitBound=1  PzUpperLimitBoundUnits=m  PzUpperLimitStiffness=1e6  PzUpperLimitStiffnessUnits=N/m  PzUpperLimitDamping=1e3  PzUpperLimitDampingUnits=N/(m/s)  PzUpperLimitTransitionRegionWidth=1e-4  PzUpperLimitTransitionRegionWidthUnits=m  PzPositionTargetSpecify=off  PzPositionTargetPriority=High  PzPositionTargetValue=0  PzPositionTargetValueUnits=m  PzVelocityTargetSpecify=off  PzVelocityTargetPriority=High  PzVelocityTargetValue=0  PzVelocityTargetValueUnits=m/s  RxEquilibriumPosition=0  RxEquilibriumPositionUnits=deg  RxSpringStiffness=0  RxSpringStiffnessUnits=N*m/deg  RxDampingCoefficient=0  RxDampingCoefficientUnits=N*m/(deg/s)  RxTorqueActuationMode=NoTorque  RxMotionActuationMode=InputMotion  RxSensePosition=off  RxSenseVelocity=off  RxSenseAcceleration=off  RxSenseTorqueForce=off  RxSenseLowerLimitTorqueForce=off  RxSenseUpperLimitTorqueForce=off  RxLowerLimitSpecify=off  RxLowerLimitBound=-90  RxLowerLimitBoundUnits=deg  RxLowerLimitStiffness=1e4  RxLowerLimitStiffnessUnits=N*m/deg  RxLowerLimitDamping=10  RxLowerLimitDampingUnits=N*m/(deg/s)  RxLowerLimitTransitionRegionWidth=0.1  RxLowerLimitTransitionRegionWidthUnits=deg  RxUpperLimitSpecify=off  RxUpperLimitBound=90  RxUpperLimitBoundUnits=deg  RxUpperLimitStiffness=1e4  RxUpperLimitStiffnessUnits=N*m/deg  RxUpperLimitDamping=10  RxUpperLimitDampingUnits=N*m/(deg/s)  RxUpperLimitTransitionRegionWidth=0.1  RxUpperLimitTransitionRegionWidthUnits=deg  RxPositionTargetSpecify=off  RxPositionTargetPriority=High  RxPositionTargetValue=0  RxPositionTargetValueUnits=deg  RxVelocityTargetSpecify=off  RxVelocityTargetPriority=High  RxVelocityTargetValue=0  RxVelocityTargetValueUnits=deg/s  RyEquilibriumPosition=0  RyEquilibriumPositionUnits=deg  RySpringStiffness=0  RySpringStiffnessUnits=N*m/deg  RyDampingCoefficient=0  RyDampingCoefficientUnits=N*m/(deg/s)  RyTorqueActuationMode=NoTorque  RyMotionActuationMode=InputMotion  RySensePosition=off  RySenseVelocity=off  RySenseAcceleration=off  RySenseTorqueForce=off  RySenseLowerLimitTorqueForce=off  RySenseUpperLimitTorqueForce=off  RyLowerLimitSpecify=off  RyLowerLimitBound=-90  RyLowerLimitBoundUnits=deg  RyLowerLimitStiffness=1e4  RyLowerLimitStiffnessUnits=N*m/deg  RyLowerLimitDamping=10  RyLowerLimitDampingUnits=N*m/(deg/s)  RyLowerLimitTransitionRegionWidth=0.1  RyLowerLimitTransitionRegionWidthUnits=deg  RyUpperLimitSpecify=off  RyUpperLimitBound=90  RyUpperLimitBoundUnits=deg  RyUpperLimitStiffness=1e4  RyUpperLimitStiffnessUnits=N*m/deg  RyUpperLimitDamping=10  RyUpperLimitDampingUnits=N*m/(deg/s)  RyUpperLimitTransitionRegionWidth=0.1  RyUpperLimitTransitionRegionWidthUnits=deg  RyPositionTargetSpecify=off  RyPositionTargetPriority=High  RyPositionTargetValue=0  RyPositionTargetValueUnits=deg  RyVelocityTargetSpecify=off  RyVelocityTargetPriority=High  RyVelocityTargetValue=0  RyVelocityTargetValueUnits=deg/s  RzEquilibriumPosition=0  RzEquilibriumPositionUnits=deg  RzSpringStiffness=0  RzSpringStiffnessUnits=N*m/deg  RzDampingCoefficient=0  RzDampingCoefficientUnits=N*m/(deg/s)  RzTorqueActuationMode=NoTorque  RzMotionActuationMode=InputMotion  RzSensePosition=off  RzSenseVelocity=off  RzSenseAcceleration=off  RzSenseTorqueForce=off  RzSenseLowerLimitTorqueForce=off  RzSenseUpperLimitTorqueForce=off  RzLowerLimitSpecify=off  RzLowerLimitBound=-90  RzLowerLimitBoundUnits=deg  RzLowerLimitStiffness=1e4  RzLowerLimitStiffnessUnits=N*m/deg  RzLowerLimitDamping=10  RzLowerLimitDampingUnits=N*m/(deg/s)  RzLowerLimitTransitionRegionWidth=0.1  RzLowerLimitTransitionRegionWidthUnits=deg  RzUpperLimitSpecify=off  RzUpperLimitBound=90  RzUpperLimitBoundUnits=deg  RzUpperLimitStiffness=1e4  RzUpperLimitStiffnessUnits=N*m/deg  RzUpperLimitDamping=10  RzUpperLimitDampingUnits=N*m/(deg/s)  RzUpperLimitTransitionRegionWidth=0.1  RzUpperLimitTransitionRegionWidthUnits=deg  RzPositionTargetSpecify=off  RzPositionTargetPriority=High  RzPositionTargetValue=0  RzPositionTargetValueUnits=deg  RzVelocityTargetSpecify=off  RzVelocityTargetPriority=High  RzVelocityTargetValue=0  RzVelocityTargetValueUnits=deg/s
      settings: SourceProductName=Simscape Multibody
  qx : Constant  Value=0
  qy : Constant  Value=0
  qz : Constant  Value=0
  F : PMIOPort  Side=Right
  B : PMIOPort  Port=2  Side=Left
  wires:
  qz/1 -> Simulink-PS Converter5/1
  Clock/1 -> Px Lookup Table/1, Pz Lookup Table/1, Py Lookup Table/1
  Py Lookup Table/1 -> Simulink-PS Converter1/1
  Pz Lookup Table/1 -> Simulink-PS Converter2/1
  Px Lookup Table/1 -> Simulink-PS Converter/1
  qx/1 -> Simulink-PS Converter3/1
  qy/1 -> Simulink-PS Converter4/1
  connections:
  Simulink-PS Converter/RConn1 -- Tool Pose/LConn2
  Simulink-PS Converter1/RConn1 -- Tool Pose/LConn3
  Simulink-PS Converter2/RConn1 -- Tool Pose/LConn4
  B/RConn1 -- Tool Pose/LConn1
  Flip Direction Rotation/RConn1 -- Tool Pose/RConn1
  Flip Direction Rotation/LConn1 -- F/RConn1
  Simulink-PS Converter5/RConn1 -- Tool Pose/LConn7
  Tool Pose/LConn5 -- Simulink-PS Converter3/RConn1
  Tool Pose/LConn6 -- Simulink-PS Converter4/RConn1

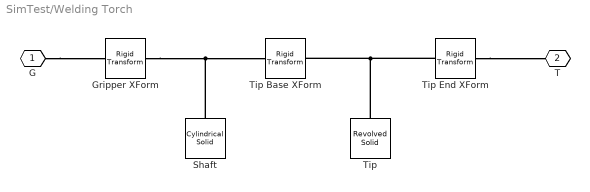
== system SimTest/Welding Torch ==
  Gripper XForm : sm_lib/Frames and Transforms/Rigid Transform  TranslationMethod=StandardAxis  TranslationStandardOffset=shaft_length / 2  TranslationLengthUnit=cm  TranslationStandardAxis=-Z  TranslationCartesianOffset=[0 0 0]  TranslationROffset=0  TranslationROffsetUnits=m  TranslationZOffset=0  TranslationZOffsetUnits=m  TranslationThetaOffset=0  TranslationThetaOffsetUnits=deg  RotationMethod=None  RotationAngleUnits=deg  RotationStandardAxis=+Z  RotationAngle=0  RotationArbitraryAxis=[0 0 1]  FollAlignAxisA=+X  BaseAlignAxisA=+Y  FollAlignAxisB=+Y  BaseAlignAxisB=+Z  RotationSequenceAxes=FollowerAxes  RotationSequence=XYX  RotationSequenceAngles=[0 0 0]  RotationSequenceAnglesUnits=deg  RotationMatrix=[1 0 0; 0 1 0; 0 0 1]
  Shaft : sm_lib/Body Elements/Cylindrical Solid  GraphicAmbientColor=[0.15 0.15 0.15 1.0]  BasedOnType=Density  CenterOfMass=[0 0 0]  CenterOfMassUnits=m  GraphicDiffuseColor=shaft_color  CylinderLength=shaft_length  CylinderLengthUnits=cm  CylinderRadius=shaft_rad  CylinderRadiusUnits=cm  Density=density  DensityUnits=kg/(m^3)  DoExposeReferenceFrame=on  GraphicEmissiveColor=[0.0 0.0 0.0 1.0]  ExportEntireGeometry=off  SerializedFrames=<Frames/>  MarkerShape=Sphere  MarkerSize=10  GraphicType=FromGeometry  InertiaType=CalculateFromGeometry  Mass=1  MassUnits=kg  MomentsOfInertia=[1 1 1]  MomentsOfInertiaUnits=kg*m^2  GraphicOpacity=1.0  ProductsOfInertia=[0 0 0]  ProductsOfInertiaUnits=kg*m^2  GraphicShininess=75  GraphicSpecularColor=[0.5 0.5 0.5 1.0]  GraphicVisPropType=SimpleVisualProperties
  Tip : sm_lib/Body Elements/Revolved Solid  GraphicAmbientColor=[0.15 0.15 0.15 1.0]  BasedOnType=Density  CenterOfMass=[0 0 0]  CenterOfMassUnits=m  GraphicDiffuseColor=tip_color  Density=density  DensityUnits=kg/(m^3)  DoExposeReferenceFrame=on  GraphicEmissiveColor=[0.0 0.0 0.0 1.0]  ExportEntireGeometry=off  SerializedFrames=<Frames/>  MarkerShape=Sphere  MarkerSize=10  GraphicType=FromGeometry  InertiaType=CalculateFromGeometry  Mass=1  MassUnits=kg  MomentsOfInertia=[1 1 1]  MomentsOfInertiaUnits=kg*m^2  GraphicOpacity=1.0  ProductsOfInertia=[0 0 0]  ProductsOfInertiaUnits=kg*m^2  RevolutionCrossSection=tip_cross_sect  RevolutionCrossSectionUnits=cm  RevolutionAngle=180  RevolutionAngleUnits=deg  RevolutionExtent=Full  GraphicShininess=75  GraphicSpecularColor=[0.5 0.5 0.5 1.0]  GraphicVisPropType=SimpleVisualProperties
      settings: SourceProductName=Simscape Multibody
  Tip Base XForm : sm_lib/Frames and Transforms/Rigid Transform  TranslationMethod=StandardAxis  TranslationStandardOffset=shaft_length / 2  TranslationLengthUnit=cm  TranslationStandardAxis=+Z  TranslationCartesianOffset=[0 0 0]  TranslationROffset=0  TranslationROffsetUnits=m  TranslationZOffset=0  TranslationZOffsetUnits=m  TranslationThetaOffset=0  TranslationThetaOffsetUnits=deg  RotationMethod=None  RotationAngleUnits=deg  RotationStandardAxis=+Z  RotationAngle=0  RotationArbitraryAxis=[0 0 1]  FollAlignAxisA=+X  BaseAlignAxisA=+Y  FollAlignAxisB=+Y  BaseAlignAxisB=+Z  RotationSequenceAxes=FollowerAxes  RotationSequence=XYX  RotationSequenceAngles=[0 0 0]  RotationSequenceAnglesUnits=deg  RotationMatrix=[1 0 0; 0 1 0; 0 0 1]
  Tip End XForm : sm_lib/Frames and Transforms/Rigid Transform  TranslationMethod=StandardAxis  TranslationStandardOffset=tip_length  TranslationLengthUnit=cm  TranslationStandardAxis=+Z  TranslationCartesianOffset=[0 0 0]  TranslationROffset=0  TranslationROffsetUnits=m  TranslationZOffset=0  TranslationZOffsetUnits=m  TranslationThetaOffset=0  TranslationThetaOffsetUnits=deg  RotationMethod=None  RotationAngleUnits=deg  RotationStandardAxis=+Z  RotationAngle=0  RotationArbitraryAxis=[0 0 1]  FollAlignAxisA=+X  BaseAlignAxisA=+Y  FollAlignAxisB=+Y  BaseAlignAxisB=+Z  RotationSequenceAxes=FollowerAxes  RotationSequence=XYX  RotationSequenceAngles=[0 0 0]  RotationSequenceAnglesUnits=deg  RotationMatrix=[1 0 0; 0 1 0; 0 0 1]
  G : PMIOPort  Side=Left
  T : PMIOPort  Port=2  Side=Right
  connections:
  Tip End XForm/LConn1 -- Tip/RConn1 -- Tip Base XForm/RConn1
  Gripper XForm/LConn1 -- Tip Base XForm/LConn1 -- Shaft/RConn1
  G/RConn1 -- Gripper XForm/RConn1
  Tip End XForm/RConn1 -- T/RConn1
